simulink model "DataDrivenRotaryPendulum"  (R2024a)
settings: Solver=ode1  StartTime=0.0  StopTime=SIMULATION_TIME  FixedStep=STEP_SIZE  MaxStep=1e-2  RelTol=1e-3  EnableMultiTasking=on
values from neighbouring files (symbols this model uses):
  Tf1 = 0.08    [dd_initialization.m]
  Tf2 = 0.08    [dd_initialization.m]
undefined symbols (not defined in the file or in its folder): kP
libraries: arduinolib x6, arduinosensorlib x2, simulink x1
settings Model: ExtModeTrigDuration=2  Creator=ikumi  LastModifiedBy=Huan
settings SolverCC: AutoInsertRateTranBlk=on
settings OptimizationCC: EnhancedBackFolding=on  PassReuseOutputArgsAs=Individual arguments  ZeroExternalMemoryAtStartup=off  ZeroInternalMemoryAtStartup=off  MaxStackSize=64  OptimizeBlockOrder=speed  DifferentSizesBufferReuse=on  OptimizationCustomize=off  EfficientTunableParamExpr=on
settings DebuggingCC: ParameterTunabilityLossMsg=error
settings HardwareCC: ProdBitPerInt=16  ProdBitPerPointer=16  ProdBitPerSizeT=16  ProdBitPerPtrDiffT=16  ProdLargestAtomicFloat=None  ProdWordSize=8  ProdHWDeviceType=Atmel->AVR
settings SFSimCC: MATLABDynamicMemAlloc=off
settings RTWCC: Description=Embedded Coder  SystemTargetFile=ert.tlc  HardwareBoard=Arduino Mega 2560  TemplateMakefile=ert_default_tmf  Toolchain=Arduino AVR  BuildConfiguration=Faster Runs
settings CodeAppCC: ForceParamTrailComments=on  IgnoreCustomStorageClasses=off  OperatorAnnotations=on  SimulinkDataObjDesc=on  SFDataObjDesc=on  InsertBlockDesc=on
settings ERTTargetCC: SupportContinuousTime=on  SupportVariableSizeSignals=on  ExtModeTransport=3  ExtModeStaticAlloc=on  ExtModeAutomaticAllocSize=off  ExtModeStaticAllocSize=2048  ExtModeMexFile=ext_xcp  ExtModeIntrfLevel=Level2 - Open

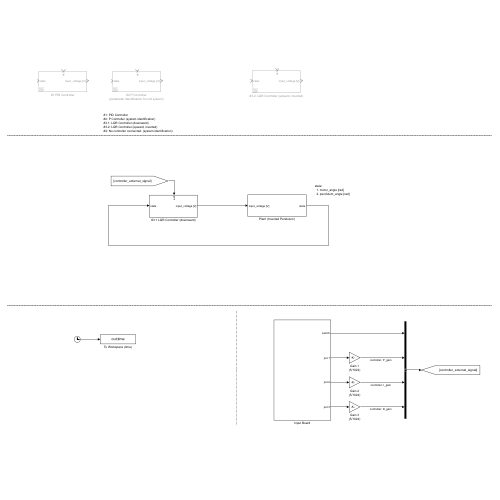
[thumbnail: Simulink's stored preview of the top-level diagram]
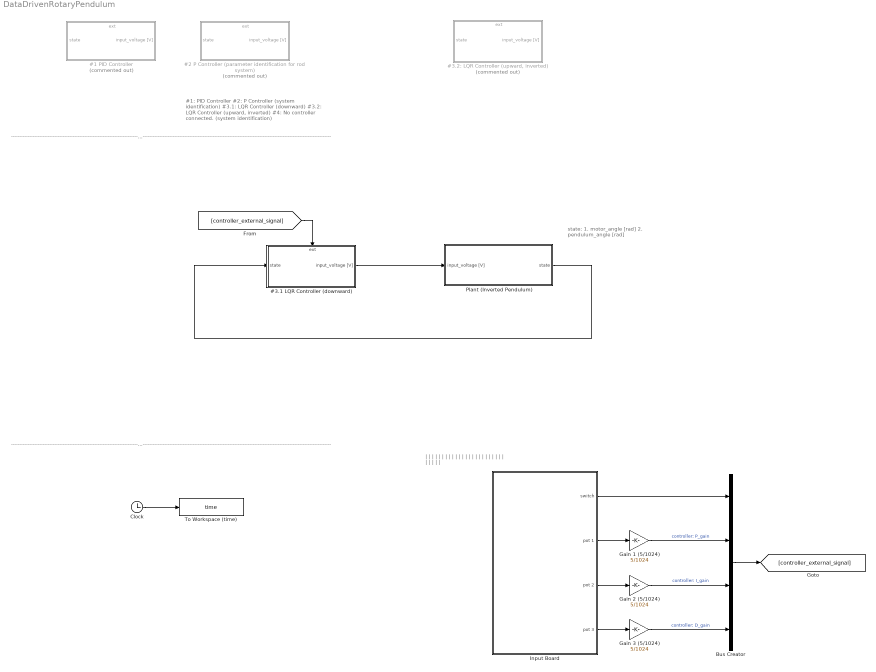
== system DataDrivenRotaryPendulum ==
  note: #1: PID Controller
      | #2: P Controller (system identification)
      | #3.1: LQR Controller (downward)
      | #3.2: LQR Controller (upward, inverted)
      | #4: No controller connected. (system identification)
  note: state:
      |   1. motor_angle [rad]
      |   2. pendulum_angle [rad]
  note: ---------------------------------------------------------------------------------------------------------------------------------------------------------------------------------------------------------------------------------------------------------------------------------------------------------------
  note: ---------------------------------------------------------------------------------------------------------------------------------------------------------------------------------------------------------------------------------------------------------------------------------------------------------------
  note: |
      | |
      | |
      | |
      | |
      | |
      | |
      | |
      | |
      | |
      | |
      | |
      | |
      | |
      | |
      | |
      | |
      | |
      | |
      | |
      | |
      | |
      | |
      | |
      | |
      | |
      | |
      | |
      | |
  #1 PID Controller : Subsystem  Commented=on
      settings: PortSchema="{\"entries\":[{\"content\":{\"sides\":[{\"content\":{\"connectorIds\":[\"In1\"]},\"type\":\"ConnectorPlacement.EquallySpacedRectSide\",\"uuid\":\"06b1af0d-78b4-43f6-add2-f1fa4860a799\"},{\"content\":{\"connectorIds\":[\"Out1\"],\"side\":\"RIGHT\"},\"type\":\"ConnectorPlacement.EquallySpacedRectSide\",\"uuid\":\"b0406211-1281-4717-b124-aa786d2c437a\"},{\"content\":{\"connectorIds\":[\"In2\"],\"side\":\"TOP\"},\"type\":\"ConnectorPlacement.EquallySpacedRectSide\",\"uuid\":\"48ff4668-84b7-46be-8f03-fa5aff98d356\"}]},\"type\":\"ConnectorPlacement.EquallySpacedConnector\",\"uuid\":\"c896c89d-b1ba-497e-85db-732d3a9a5cce\"}],\"packageUris\":[\"http://schema.mathworks.com/mf0/Connector/R2020b\"],\"version\":\"1.0\"}"
  #2 P Controller (parameter identification for rod system) : Subsystem  Commented=on
      settings: PortSchema="{\"entries\":[{\"content\":{\"sides\":[{\"content\":{\"connectorIds\":[\"In1\"]},\"type\":\"ConnectorPlacement.EquallySpacedRectSide\",\"uuid\":\"06b1af0d-78b4-43f6-add2-f1fa4860a799\"},{\"content\":{\"connectorIds\":[\"Out1\"],\"side\":\"RIGHT\"},\"type\":\"ConnectorPlacement.EquallySpacedRectSide\",\"uuid\":\"b0406211-1281-4717-b124-aa786d2c437a\"},{\"content\":{\"connectorIds\":[\"In2\"],\"side\":\"TOP\"},\"type\":\"ConnectorPlacement.EquallySpacedRectSide\",\"uuid\":\"48ff4668-84b7-46be-8f03-fa5aff98d356\"}]},\"type\":\"ConnectorPlacement.EquallySpacedConnector\",\"uuid\":\"c896c89d-b1ba-497e-85db-732d3a9a5cce\"}],\"packageUris\":[\"http://schema.mathworks.com/mf0/Connector/R2020b\"],\"version\":\"1.0\"}"
  #3.1 LQR Controller (downward) : Subsystem
      settings: PortSchema="{\"entries\":[{\"content\":{\"sides\":[{\"content\":{\"connectorIds\":[\"In1\"]},\"type\":\"ConnectorPlacement.EquallySpacedRectSide\",\"uuid\":\"b3e4cd4f-c8f8-4ac1-a1f2-23e37a640ad8\"},{\"content\":{\"connectorIds\":[\"Out1\"],\"side\":\"RIGHT\"},\"type\":\"ConnectorPlacement.EquallySpacedRectSide\",\"uuid\":\"02360ac2-7779-4092-8f90-91424c435481\"},{\"content\":{\"connectorIds\":[\"In2\"],\"side\":\"TOP\"},\"type\":\"ConnectorPlacement.EquallySpacedRectSide\",\"uuid\":\"f86ccd1f-d9a7-4ad2-ba4f-ea0c1bd32c00\"}]},\"type\":\"ConnectorPlacement.EquallySpacedConnector\",\"uuid\":\"875a99af-631d-422d-8b23-87ab8d1e3283\"}],\"packageUris\":[\"http://schema.mathworks.com/mf0/Connector/R2020b\"],\"version\":\"1.0\"}"
  "#3.2: LQR Controller (upward, inverted)" : Subsystem  Commented=on
      settings: PortSchema="{\"entries\":[{\"content\":{\"sides\":[{\"content\":{\"connectorIds\":[\"In1\"]},\"type\":\"ConnectorPlacement.EquallySpacedRectSide\",\"uuid\":\"b3e4cd4f-c8f8-4ac1-a1f2-23e37a640ad8\"},{\"content\":{\"connectorIds\":[\"Out1\"],\"side\":\"RIGHT\"},\"type\":\"ConnectorPlacement.EquallySpacedRectSide\",\"uuid\":\"02360ac2-7779-4092-8f90-91424c435481\"},{\"content\":{\"connectorIds\":[\"In2\"],\"side\":\"TOP\"},\"type\":\"ConnectorPlacement.EquallySpacedRectSide\",\"uuid\":\"f86ccd1f-d9a7-4ad2-ba4f-ea0c1bd32c00\"}]},\"type\":\"ConnectorPlacement.EquallySpacedConnector\",\"uuid\":\"875a99af-631d-422d-8b23-87ab8d1e3283\"}],\"packageUris\":[\"http://schema.mathworks.com/mf0/Connector/R2020b\"],\"version\":\"1.0\"}"
  Bus Creator : BusCreator  Inputs=4
  Clock : Clock
  Gain 1 (5/1024) : Gain  Gain=5/1024
  Gain 2 (5/1024) : Gain  Gain=5/1024
  Gain 3 (5/1024) : Gain  Gain=5/1024
  Input Board : Subsystem
  Plant (Inverted Pendulum) : Subsystem
  To Workspace (time) : ToWorkspace  VariableName=time  SaveFormat=Timeseries  SampleTime=-1
  wires:
  #3.1 LQR Controller (downward)/1(input_voltage [V]) -> Plant (Inverted Pendulum)/1(input_voltage [V])
  Input Board/1(switch) -> Bus Creator/1
  Gain 2 (5/1024)/1 -> Bus Creator/3  "controller: I_gain"
  Input Board/4(pot 3) -> Gain 3 (5/1024)/1
  Gain 1 (5/1024)/1 -> Bus Creator/2  "controller: P_gain"
  Gain 3 (5/1024)/1 -> Bus Creator/4  "controller: D_gain"
  Input Board/3(pot 2) -> Gain 2 (5/1024)/1
  Input Board/2(pot 1) -> Gain 1 (5/1024)/1
  Bus Creator/1 -> [controller_external_signal]
  [controller_external_signal] -> #3.1 LQR Controller (downward)/2(ext)
  Clock/1 -> To Workspace (time)/1
  Plant (Inverted Pendulum)/1(state) -> #3.1 LQR Controller (downward)/1(state)

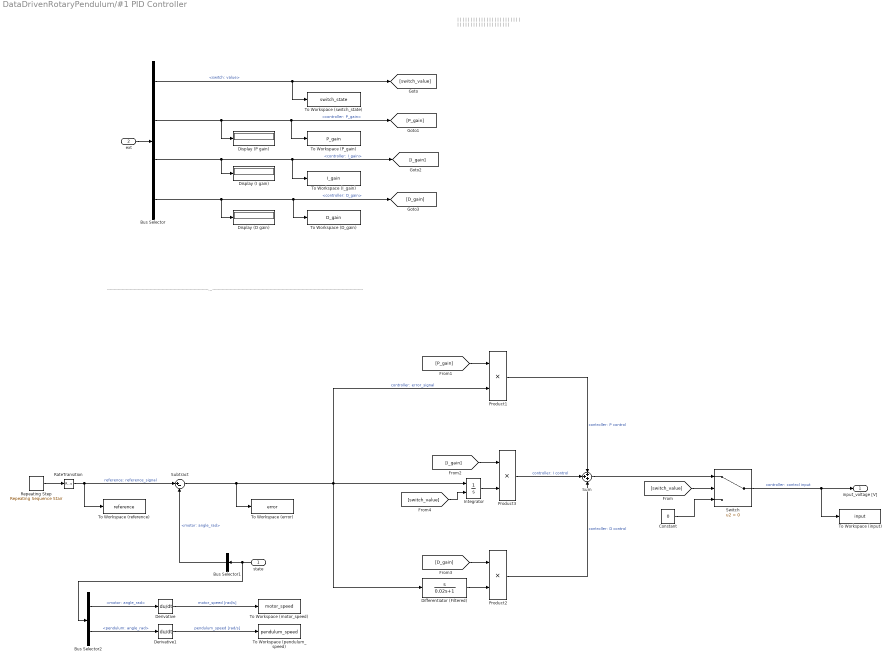
== system DataDrivenRotaryPendulum/#1 PID Controller ==
  note: ---------------------------------------------------------------------------------------------------------------------------------------------------------------------------------------------------------------------------------------------------------------------------------------------------------------
  note: |
      | |
      | |
      | |
      | |
      | |
      | |
      | |
      | |
      | |
      | |
      | |
      | |
      | |
      | |
      | |
      | |
      | |
      | |
      | |
      | |
      | |
      | |
      | |
      | |
      | |
      | |
      | |
      | |
      | |
      | |
      | |
      | |
      | |
      | |
      | |
      | |
      | |
      | |
      | |
      | |
      | |
      | |
      | |
  state : Inport
  ext : Inport  Port=2
  " Integrator " : Integrator  ExternalReset=rising
  Bus Selector : BusSelector  OutputSignals=switch: value,controller: P_gain,controller: I_gain,controller: D_gain
  Bus Selector1 : BusSelector  OutputSignals=motor: angle_rad
  Bus Selector2 : BusSelector  OutputSignals=motor: angle_rad,pendulum: angle_rad
  Constant : Constant  Value=0
  Derivative : Derivative
  Derivative1 : Derivative
  Differentiator (Filtered) : TransferFcn  Numerator=[1 0]  Denominator=[0.02 1]
  Display (D gain) : Display
  Display (I gain) : Display
  Display (P gain) : Display
  Product1 : Product
  Product2 : Product
  Product3 : Product
  RateTransition : RateTransition  OutPortSampleTime=STEP_SIZE
  Repeating Step : simulink/Sources/Repeating Sequence Stair  OutValues=[pi/2 0 -pi/2 0]  tsamp=2.5  OutMin=[]  OutMax=[]  OutDataTypeStr=double  OutputDataTypeScalingMode=double  OutDataType=fixdt(0,8)  ConRadixGroup=Best Precision: Vector-wise  OutScaling=2^-12
  Subtract : Sum  Inputs=|+-
  Sum : Sum  Inputs=+++
  Switch : Switch  Criteria=u2 > Threshold  SaturateOnIntegerOverflow=off  InputSameDT=off
  To Workspace (D_gain) : ToWorkspace  VariableName=D_gain  SaveFormat=Timeseries  SampleTime=-1
  To Workspace (I_gain) : ToWorkspace  VariableName=I_gain  SaveFormat=Timeseries  SampleTime=-1
  To Workspace (P_gain) : ToWorkspace  VariableName=P_gain  SaveFormat=Timeseries  SampleTime=-1
  To Workspace (error) : ToWorkspace  VariableName=error  SaveFormat=Timeseries  SampleTime=-1
  To Workspace (input) : ToWorkspace  VariableName=input  SaveFormat=Timeseries  SampleTime=-1
  To Workspace (motor_speed) : ToWorkspace  VariableName=motor_speed  SaveFormat=Timeseries  SampleTime=-1
  To Workspace (pendulum_speed) : ToWorkspace  VariableName=pendulum_speed  SaveFormat=Timeseries  SampleTime=-1
  To Workspace (reference) : ToWorkspace  VariableName=reference  SaveFormat=Timeseries  SampleTime=-1
  To Workspace (switch_state) : ToWorkspace  VariableName=switch_state  SaveFormat=Timeseries  SampleTime=-1
  input_voltage [V] : Outport
  wires:
  Constant/1 -> Switch/3
  Subtract/1 -> To Workspace (error)/1, Differentiator (Filtered)/1, " Integrator "/1, Product1/2  "controller: error_signal"
  [P_gain] -> Product1/1
  [I_gain] -> Product3/1
  [D_gain] -> Product2/1
  " Integrator "/1 -> Product3/2
  Differentiator (Filtered)/1 -> Product2/2
  Product3/1 -> Sum/2  "controller: I control"
  Product2/1 -> Sum/3  "controller: D control"
  Product1/1 -> Sum/1  "controller: P control"
  Sum/1 -> Switch/1
  [switch_value] -> Switch/2
  Switch/1 -> To Workspace (input)/1, input_voltage [V]/1  "controller: control input"
  [switch_value] -> " Integrator "/2
  Bus Selector/3 -> To Workspace (I_gain)/1, [I_gain], Display (I gain)/1  "<controller: I_gain>"
  Bus Selector/4 -> To Workspace (D_gain)/1, [D_gain], Display (D gain)/1  "<controller: D_gain>"
  Bus Selector/1 -> To Workspace (switch_state)/1, [switch_value]  "<switch: value>"
  Bus Selector/2 -> To Workspace (P_gain)/1, [P_gain], Display (P gain)/1  "<controller: P_gain>"
  ext/1 -> Bus Selector/1
  Repeating Step/1 -> RateTransition/1
  RateTransition/1 -> Subtract/1, To Workspace (reference)/1  "reference: reference_signal"
  Bus Selector1/1 -> Subtract/2  "<motor: angle_rad>"
  Bus Selector2/2 -> Derivative1/1  "<pendulum: angle_rad>"
  Derivative1/1 -> To Workspace (pendulum_speed)/1  "pendulum_speed [rad/s]"
  state/1 -> Bus Selector2/1, Bus Selector1/1
  Bus Selector2/1 -> Derivative/1  "<motor: angle_rad>"
  Derivative/1 -> To Workspace (motor_speed)/1  "motor_speed [rad/s]"

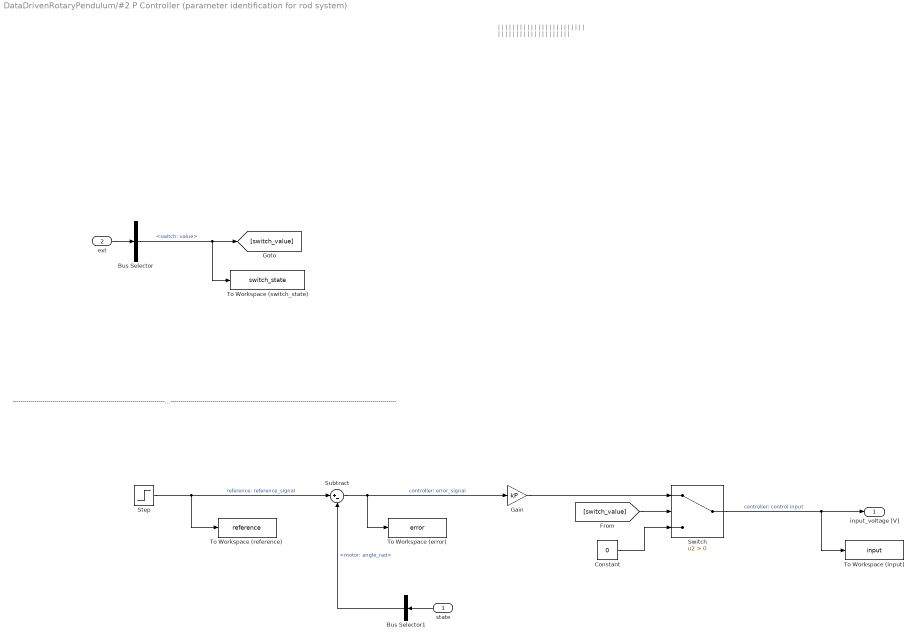
== system DataDrivenRotaryPendulum/#2 P Controller (parameter identification for rod system) ==
  note: ---------------------------------------------------------------------------------------------------------------------------------------------------------------------------------------------------------------------------------------------------------------------------------------------------------------
  note: |
      | |
      | |
      | |
      | |
      | |
      | |
      | |
      | |
      | |
      | |
      | |
      | |
      | |
      | |
      | |
      | |
      | |
      | |
      | |
      | |
      | |
      | |
      | |
      | |
      | |
      | |
      | |
      | |
      | |
      | |
      | |
      | |
      | |
      | |
      | |
      | |
      | |
      | |
      | |
      | |
      | |
      | |
      | |
  state : Inport
  ext : Inport  Port=2
  Bus Selector : BusSelector  OutputSignals=switch: value
  Bus Selector1 : BusSelector  OutputSignals=motor: angle_rad
  Constant : Constant  Value=0
  Gain : Gain  Gain=kP
  Step : Step  After=pi/2  SampleTime=0
  Subtract : Sum  Inputs=|+-
  Switch : Switch  Criteria=u2 > Threshold  SaturateOnIntegerOverflow=off  InputSameDT=off
  To Workspace (error) : ToWorkspace  VariableName=error  SaveFormat=Timeseries  SampleTime=-1
  To Workspace (input) : ToWorkspace  VariableName=input  SaveFormat=Timeseries  SampleTime=-1
  To Workspace (reference) : ToWorkspace  VariableName=reference  SaveFormat=Timeseries  SampleTime=-1
  To Workspace (switch_state) : ToWorkspace  VariableName=switch_state  SaveFormat=Timeseries  SampleTime=-1
  input_voltage [V] : Outport
  wires:
  Constant/1 -> Switch/3
  Subtract/1 -> Gain/1, To Workspace (error)/1  "controller: error_signal"
  Gain/1 -> Switch/1
  [switch_value] -> Switch/2
  Switch/1 -> To Workspace (input)/1, input_voltage [V]/1  "controller: control input"
  Bus Selector/1 -> [switch_value], To Workspace (switch_state)/1  "<switch: value>"
  ext/1 -> Bus Selector/1
  Step/1 -> Subtract/1, To Workspace (reference)/1  "reference: reference_signal"
  state/1 -> Bus Selector1/1
  Bus Selector1/1 -> Subtract/2  "<motor: angle_rad>"

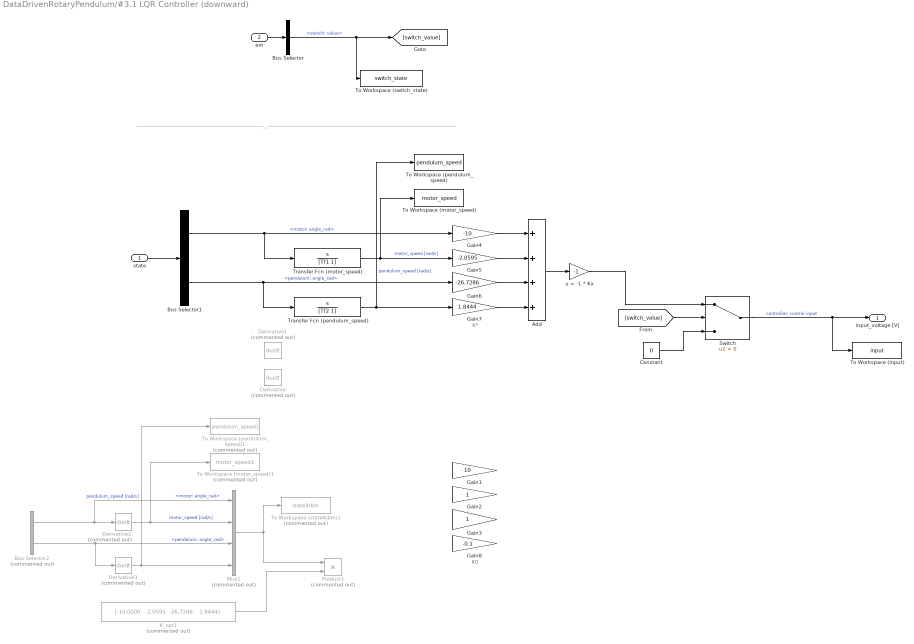
== system DataDrivenRotaryPendulum/#3.1 LQR Controller (downward) ==
  note: ---------------------------------------------------------------------------------------------------------------------------------------------------------------------------------------------------------------------------------------------------------------------------------------------------------------
  note: K*
  note: K0
  state : Inport
  ext : Inport  Port=2
  Add : Sum  Inputs=++++
  Bus Selector : BusSelector  OutputSignals=switch: value
  Bus Selector1 : BusSelector  OutputSignals=motor: angle_rad,pendulum: angle_rad
  Bus Selector2 : BusSelector  Commented=on  OutputSignals=motor: angle_rad,pendulum: angle_rad
  Constant : Constant  Value=0
  Derivative{,1..3} (4 alike) : Derivative  Commented=on
  Gain1 : Gain  Gain=10
  Gain2 : Gain
  Gain3 : Gain
  Gain4 : Gain  Gain=-10
  Gain5 : Gain  Gain=-2.0595
  Gain6 : Gain  Gain=-26.7286
  Gain7 : Gain  Gain=1.8444
  Gain8 : Gain  Gain=-0.1
  K_opt1 : Constant  Commented=on  Value="[-10.0000   -2.0595  -26.7286    1.8444]"
  Mux1 : Mux  Commented=on
  Product1 : Product  Commented=on
  Switch : Switch  Criteria=u2 > Threshold  SaturateOnIntegerOverflow=off  InputSameDT=off
  To Workspace (input) : ToWorkspace  VariableName=input  SaveFormat=Timeseries  SampleTime=-1
  To Workspace (motor_speed) : ToWorkspace  VariableName=motor_speed  SaveFormat=Timeseries  SampleTime=-1
  To Workspace (motor_speed)1 : ToWorkspace  Commented=on  VariableName=motor_speed1  SaveFormat=Timeseries  SampleTime=-1
  To Workspace (pendulum_speed) : ToWorkspace  VariableName=pendulum_speed  SaveFormat=Timeseries  SampleTime=-1
  To Workspace (pendulum_speed)1 : ToWorkspace  Commented=on  VariableName=pendulum_speed1  SaveFormat=Timeseries  SampleTime=-1
  To Workspace (state4dim)1 : ToWorkspace  Commented=on  VariableName=state4dim  SaveFormat=Timeseries  SampleTime=-1
  To Workspace (switch_state) : ToWorkspace  VariableName=switch_state  SaveFormat=Timeseries  SampleTime=-1
  "Transfer Fcn (motor_speed) " : TransferFcn  Numerator=[1 0]  Denominator=[Tf1 1]
  Transfer Fcn (pendulum_speed) : TransferFcn  Numerator=[1 0]  Denominator=[Tf2 1]
  u = -1 * Kx : Gain  Gain=-1
  input_voltage [V] : Outport
  wires:
  Constant/1 -> Switch/3
  [switch_value] -> Switch/2
  Switch/1 -> To Workspace (input)/1, input_voltage [V]/1  "controller: control input"
  state/1 -> Bus Selector1/1
  Bus Selector1/1 -> Gain4/1, "Transfer Fcn (motor_speed) "/1  "<motor: angle_rad>"
  Bus Selector1/2 -> Gain6/1, Transfer Fcn (pendulum_speed)/1  "<pendulum: angle_rad>"
  "Transfer Fcn (motor_speed) "/1 -> Gain5/1, To Workspace (motor_speed)/1  "motor_speed [rad/s]"
  Transfer Fcn (pendulum_speed)/1 -> Gain7/1, To Workspace (pendulum_speed)/1  "pendulum_speed [rad/s]"
  Add/1 -> u = -1 * Kx/1
  Bus Selector/1 -> [switch_value], To Workspace (switch_state)/1  "<switch: value>"
  ext/1 -> Bus Selector/1
  Bus Selector2/2 -> Derivative3/1, Mux1/3  "<pendulum: angle_rad>"
  Mux1/1 -> To Workspace (state4dim)1/1, Product1/1
  Derivative3/1 -> To Workspace (pendulum_speed)1/1, Mux1/4  "pendulum_speed [rad/s]"
  K_opt1/1 -> Product1/2
  Bus Selector2/1 -> Mux1/1, Derivative2/1  "<motor: angle_rad>"
  Derivative2/1 -> To Workspace (motor_speed)1/1, Mux1/2  "motor_speed [rad/s]"
  Gain4/1 -> Add/1
  Gain5/1 -> Add/2
  Gain6/1 -> Add/3
  Gain7/1 -> Add/4
  u = -1 * Kx/1 -> Switch/1

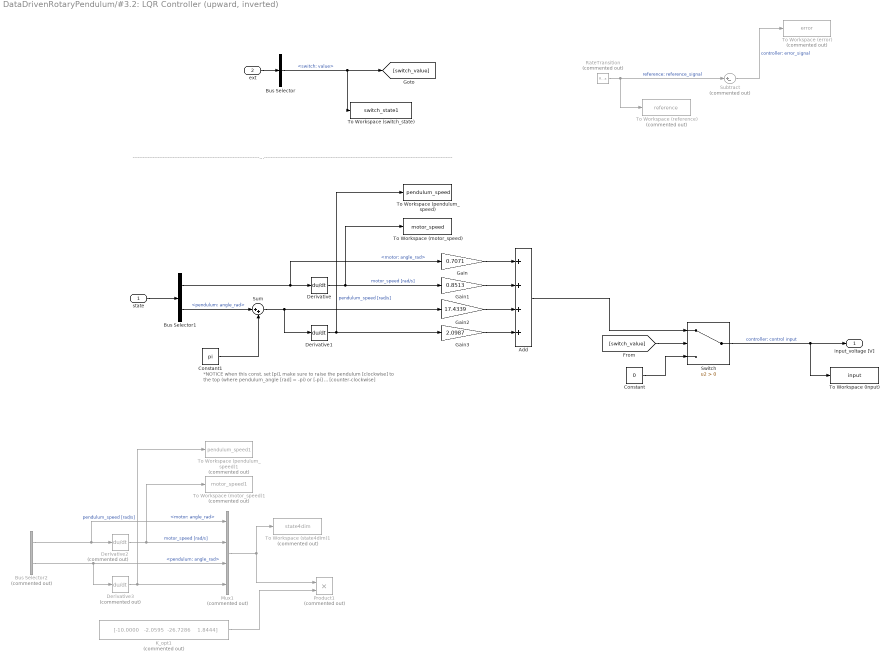
== system DataDrivenRotaryPendulum/#3.2: LQR Controller (upward, inverted) ==
  note: *NOTICE
      | when this const. set [pi], make sure to
      | raise the pendulum [clockwise] to the top (where pendulum_angle [rad] = -pi)
      | or [-pi] ... [counter-clockwise]
  note: ---------------------------------------------------------------------------------------------------------------------------------------------------------------------------------------------------------------------------------------------------------------------------------------------------------------
  state : Inport
  ext : Inport  Port=2
  Add : Sum  Inputs=++++
  Bus Selector : BusSelector  OutputSignals=switch: value
  Bus Selector1 : BusSelector  OutputSignals=motor: angle_rad,pendulum: angle_rad
  Bus Selector2 : BusSelector  Commented=on  OutputSignals=motor: angle_rad,pendulum: angle_rad
  Constant : Constant  Value=0
  Constant1 : Constant  Value=pi
  Derivative : Derivative
  Derivative1 : Derivative
  Derivative2 : Derivative  Commented=on
  Derivative3 : Derivative  Commented=on
  Gain : Gain  Gain=0.7071
  Gain1 : Gain  Gain=0.8513
  Gain2 : Gain  Gain=17.4339
  Gain3 : Gain  Gain=2.0987
  K_opt1 : Constant  Commented=on  Value="[-10.0000   -2.0595  -26.7286    1.8444]"
  Mux1 : Mux  Commented=on
  Product1 : Product  Commented=on
  RateTransition : RateTransition  Commented=on  OutPortSampleTime=STEP_SIZE
  Subtract : Sum  Commented=on  Inputs=|+-
  Sum : Sum  Inputs=|++
  Switch : Switch  Criteria=u2 > Threshold  SaturateOnIntegerOverflow=off  InputSameDT=off
  To Workspace (error) : ToWorkspace  Commented=on  VariableName=error  SaveFormat=Timeseries  SampleTime=-1
  To Workspace (input) : ToWorkspace  VariableName=input  SaveFormat=Timeseries  SampleTime=-1
  To Workspace (motor_speed) : ToWorkspace  VariableName=motor_speed  SaveFormat=Timeseries  SampleTime=-1
  To Workspace (motor_speed)1 : ToWorkspace  Commented=on  VariableName=motor_speed1  SaveFormat=Timeseries  SampleTime=-1
  To Workspace (pendulum_speed) : ToWorkspace  VariableName=pendulum_speed  SaveFormat=Timeseries  SampleTime=-1
  To Workspace (pendulum_speed)1 : ToWorkspace  Commented=on  VariableName=pendulum_speed1  SaveFormat=Timeseries  SampleTime=-1
  To Workspace (reference) : ToWorkspace  Commented=on  VariableName=reference  SaveFormat=Timeseries  SampleTime=-1
  To Workspace (state4dim)1 : ToWorkspace  Commented=on  VariableName=state4dim  SaveFormat=Timeseries  SampleTime=-1
  To Workspace (switch_state) : ToWorkspace  VariableName=switch_state1  SaveFormat=Timeseries  SampleTime=-1
  input_voltage [V] : Outport
  wires:
  Sum/1 -> Gain2/1, Derivative1/1
  Constant1/1 -> Sum/2
  Gain3/1 -> Add/4
  Gain2/1 -> Add/3
  Gain1/1 -> Add/2
  Gain/1 -> Add/1
  Derivative2/1 -> Mux1/2, To Workspace (motor_speed)1/1  "motor_speed [rad/s]"
  Bus Selector2/1 -> Derivative2/1, Mux1/1  "<motor: angle_rad>"
  K_opt1/1 -> Product1/2
  Derivative3/1 -> Mux1/4, To Workspace (pendulum_speed)1/1  "pendulum_speed [rad/s]"
  Mux1/1 -> Product1/1, To Workspace (state4dim)1/1
  Bus Selector2/2 -> Mux1/3, Derivative3/1  "<pendulum: angle_rad>"
  ext/1 -> Bus Selector/1
  Bus Selector/1 -> To Workspace (switch_state)/1, [switch_value]  "<switch: value>"
  Add/1 -> Switch/1
  Derivative1/1 -> Gain3/1, To Workspace (pendulum_speed)/1  "pendulum_speed [rad/s]"
  Derivative/1 -> Gain1/1, To Workspace (motor_speed)/1  "motor_speed [rad/s]"
  Bus Selector1/2 -> Sum/1  "<pendulum: angle_rad>"
  Bus Selector1/1 -> Gain/1, Derivative/1  "<motor: angle_rad>"
  state/1 -> Bus Selector1/1
  RateTransition/1 -> To Workspace (reference)/1, Subtract/1  "reference: reference_signal"
  Switch/1 -> input_voltage [V]/1, To Workspace (input)/1  "controller: control input"
  [switch_value] -> Switch/2
  Subtract/1 -> To Workspace (error)/1  "controller: error_signal"
  Constant/1 -> Switch/3

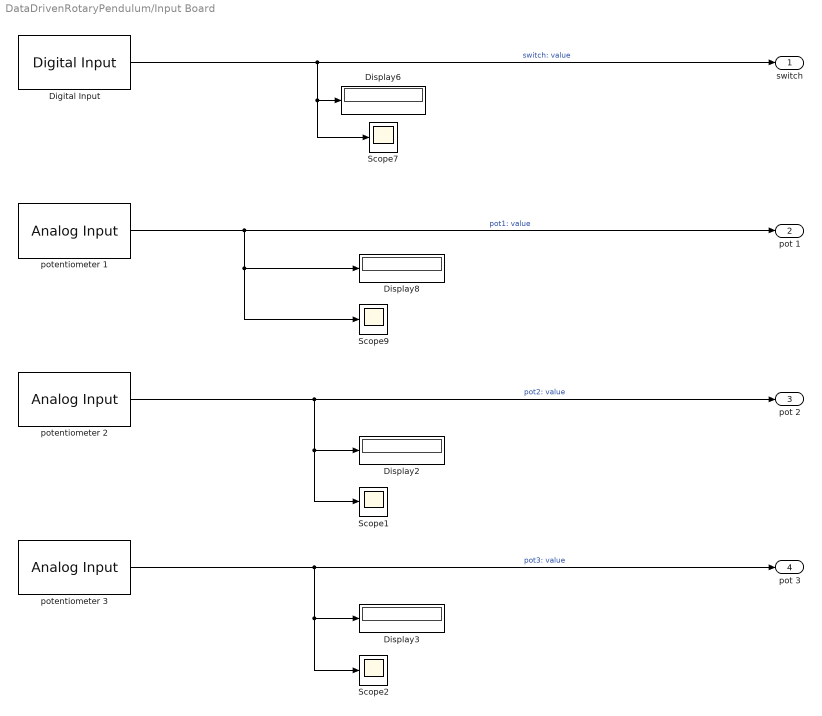
== system DataDrivenRotaryPendulum/Input Board ==
  Digital Input : arduinolib/Digital Input  pinNumber=8  mode=Default  Direction=input  SampleTime=-1  blockPlatform=arduino
  Display{2..3,6,8} (4 alike) : Display
  Scope{1..2,7,9} (4 alike) : Scope
  potentiometer 1 : arduinolib/Analog Input  pinNumber=0  ReadResultsOnly=off  ConversionTriggerSource=Software  ExternalTriggerType=uint32( 0 )  OutputDataType=uint16  EnableConversionCompleteNotify=off  EnableOuputStatus=off  SampleTime=-1  blockPlatform=arduino
  potentiometer 2 : arduinolib/Analog Input  pinNumber=1  ReadResultsOnly=off  ConversionTriggerSource=Software  ExternalTriggerType=uint32( 0 )  OutputDataType=uint16  EnableConversionCompleteNotify=off  EnableOuputStatus=off  SampleTime=-1  blockPlatform=arduino
  potentiometer 3 : arduinolib/Analog Input  pinNumber=2  ReadResultsOnly=off  ConversionTriggerSource=Software  ExternalTriggerType=uint32( 0 )  OutputDataType=uint16  EnableConversionCompleteNotify=off  EnableOuputStatus=off  SampleTime=-1  blockPlatform=arduino
  switch : Outport
  pot 1 : Outport  Port=2
  pot 2 : Outport  Port=3
  pot 3 : Outport  Port=4
  wires:
  Digital Input/1 -> switch/1, Scope7/1, Display6/1  "switch: value"
  potentiometer 3/1 -> pot 3/1, Scope2/1, Display3/1  "pot3: value"
  potentiometer 2/1 -> pot 2/1, Scope1/1, Display2/1  "pot2: value"
  potentiometer 1/1 -> Scope9/1, Display8/1, pot 1/1  "pot1: value"

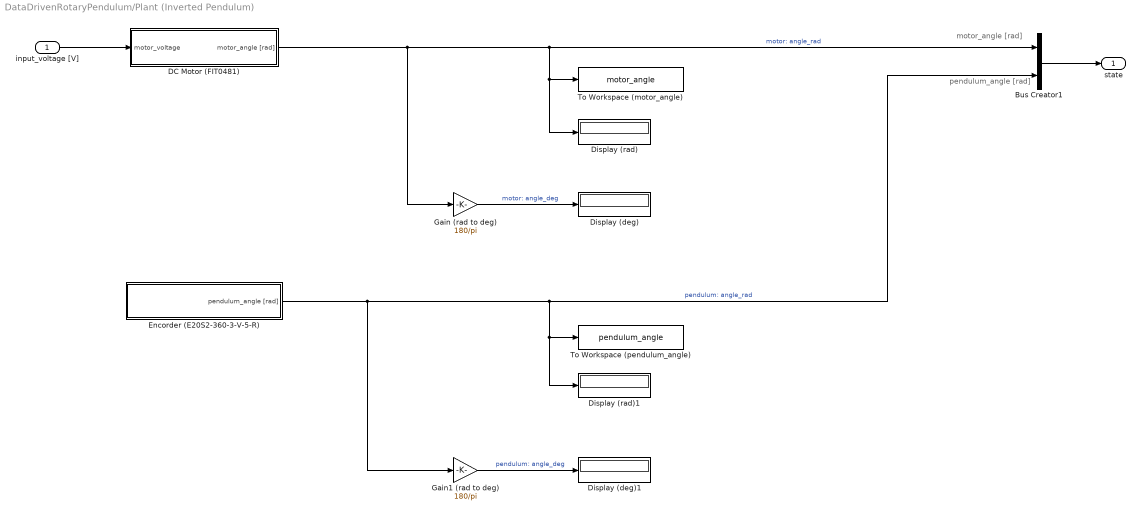
== system DataDrivenRotaryPendulum/Plant (Inverted Pendulum) ==
  note: pendulum_angle [rad]
  note: motor_angle [rad]
  input_voltage [V] : Inport
  Bus Creator1 : BusCreator  Inputs=2
  DC Motor (FIT0481) : Subsystem
  Display (deg) : Display
  Display (deg)1 : Display
  Display (rad) : Display
  Display (rad)1 : Display
  Encorder (E20S2-360-3-V-5-R) : Subsystem
  Gain (rad to deg) : Gain  Gain=180/pi
  Gain1 (rad to deg) : Gain  Gain=180/pi
  To Workspace (motor_angle) : ToWorkspace  VariableName=motor_angle  SaveFormat=Timeseries  SampleTime=-1
  To Workspace (pendulum_angle) : ToWorkspace  VariableName=pendulum_angle  SaveFormat=Timeseries  SampleTime=-1
  state : Outport
  wires:
  DC Motor (FIT0481)/1(motor_angle [rad]) -> To Workspace (motor_angle)/1, Display (rad)/1, Bus Creator1/1, Gain (rad to deg)/1  "motor: angle_rad"
  Gain (rad to deg)/1 -> Display (deg)/1  "motor: angle_deg"
  input_voltage [V]/1 -> DC Motor (FIT0481)/1(motor_voltage)
  Encorder (E20S2-360-3-V-5-R)/1(pendulum_angle [rad]) -> Bus Creator1/2, To Workspace (pendulum_angle)/1, Display (rad)1/1, Gain1 (rad to deg)/1  "pendulum: angle_rad"
  Gain1 (rad to deg)/1 -> Display (deg)1/1  "pendulum: angle_deg"
  Bus Creator1/1 -> state/1

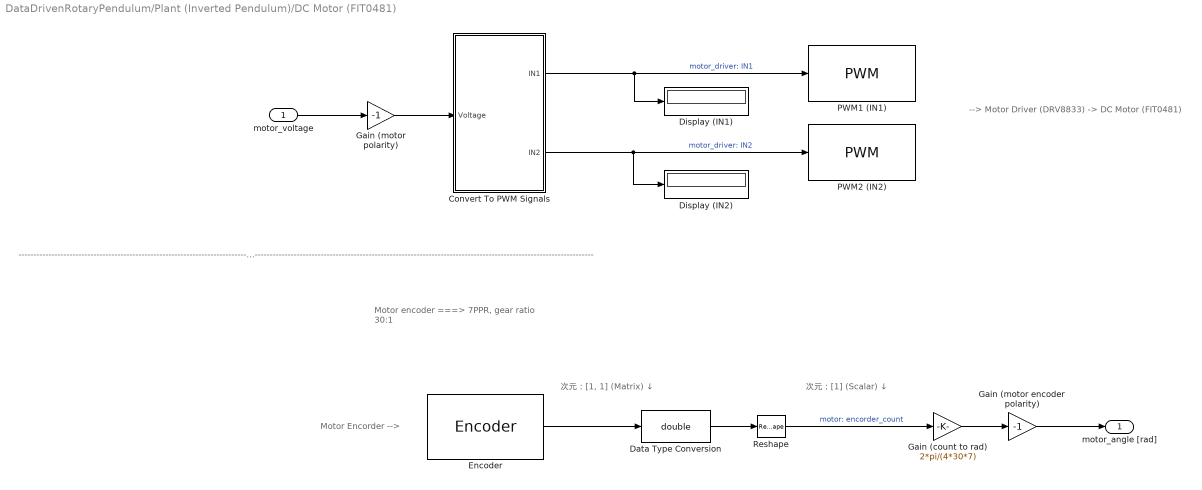
== system DataDrivenRotaryPendulum/Plant (Inverted Pendulum)/DC Motor (FIT0481) ==
  note: Motor Encorder -->
  note: --> Motor Driver (DRV8833) -> DC Motor (FIT0481)
  note: Motor encoder
      | ===> 7PPR, gear ratio 30:1
  note: 次元：[1, 1] (Matrix)
      | ↓
  note: 次元：[1] (Scalar)
      | ↓
  note: ---------------------------------------------------------------------------------------------------------------------------------------------------------------------------------------------------------------------------------------------------------------------------------------------------------------
  motor_voltage : Inport
  Convert To PWM Signals : Subsystem
  Data Type Conversion : DataTypeConversion  OutDataTypeStr=double  SaturateOnIntegerOverflow=off  RndMeth=Floor
  Display (IN1) : Display
  Display (IN2) : Display
  Encoder : arduinosensorlib/Encoder  InputA=2  InputB=3  Mode=No reset  SampleTime=-1
  Gain (count to rad) : Gain  Gain=2*pi/(4*30*7)
  Gain (motor encoder polarity) : Gain  Gain=-1
  Gain (motor polarity) : Gain  Gain=-1
  PWM1 (IN1) : arduinolib/PWM  pinNumber=6  frequencyType=Default  desiredFrequency=490.2  achievableFrequency=490.2
  PWM2 (IN2) : arduinolib/PWM  pinNumber=7  frequencyType=Default  desiredFrequency=490.2  achievableFrequency=490.2
  Reshape : Reshape
  motor_angle [rad] : Outport
  wires:
  Gain (motor polarity)/1 -> Convert To PWM Signals/1(Voltage)
  Convert To PWM Signals/1(IN1) -> Display (IN1)/1, PWM1 (IN1)/1  "motor_driver: IN1"
  Convert To PWM Signals/2(IN2) -> Display (IN2)/1, PWM2 (IN2)/1  "motor_driver: IN2"
  Encoder/1 -> Data Type Conversion/1
  Gain (count to rad)/1 -> Gain (motor encoder polarity)/1
  Reshape/1 -> Gain (count to rad)/1  "motor: encorder_count"
  Data Type Conversion/1 -> Reshape/1
  Gain (motor encoder polarity)/1 -> motor_angle [rad]/1
  motor_voltage/1 -> Gain (motor polarity)/1

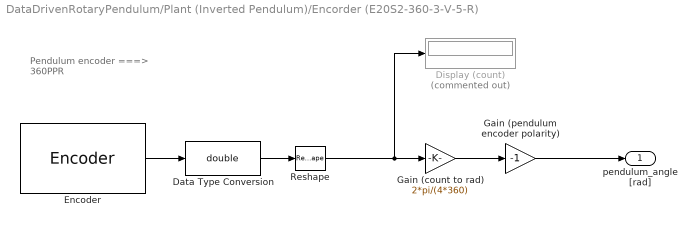
== system DataDrivenRotaryPendulum/Plant (Inverted Pendulum)/Encorder (E20S2-360-3-V-5-R) ==
  note: Pendulum encoder
      | ===> 360PPR
  Data Type Conversion : DataTypeConversion  OutDataTypeStr=double  SaturateOnIntegerOverflow=off  RndMeth=Floor
  Display (count) : Display  Commented=on
  Encoder : arduinosensorlib/Encoder  InputA=18  InputB=19  Mode=No reset  SampleTime=-1
  Gain (count to rad) : Gain  Gain=2*pi/(4*360)
  Gain (pendulum encoder polarity) : Gain  Gain=-1
  Reshape : Reshape
  pendulum_angle [rad] : Outport
  wires:
  Data Type Conversion/1 -> Reshape/1
  Reshape/1 -> Display (count)/1, Gain (count to rad)/1
  Gain (pendulum encoder polarity)/1 -> pendulum_angle [rad]/1
  Gain (count to rad)/1 -> Gain (pendulum encoder polarity)/1
  Encoder/1 -> Data Type Conversion/1

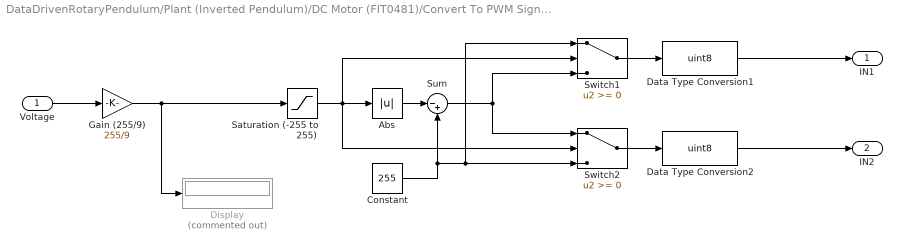
== system DataDrivenRotaryPendulum/Plant (Inverted Pendulum)/DC Motor (FIT0481)/Convert To PWM Signals ==
  Voltage : Inport
  Abs : Abs  SaturateOnIntegerOverflow=off
  Constant : Constant  Value=255  SampleTime=-1
  Data Type Conversion1 : DataTypeConversion  OutDataTypeStr=uint8  SaturateOnIntegerOverflow=off  RndMeth=Floor
  Data Type Conversion2 : DataTypeConversion  OutDataTypeStr=uint8  SaturateOnIntegerOverflow=off  RndMeth=Floor
  Display : Display  Commented=on
  Gain (255/9) : Gain  Gain=255/9
  Saturation (-255 to 255) : Saturate  UpperLimit=255  LowerLimit=-255
  Sum : Sum  Inputs=|-+
  Switch1 : Switch  SaturateOnIntegerOverflow=off  InputSameDT=off
  Switch2 : Switch  SaturateOnIntegerOverflow=off  InputSameDT=off
  IN1 : Outport
  IN2 : Outport  Port=2
  wires:
  Gain (255/9)/1 -> Display/1, Saturation (-255 to 255)/1
  Voltage/1 -> Gain (255/9)/1
  Abs/1 -> Sum/1
  Sum/1 -> Switch2/1, Switch1/3
  Switch2/1 -> Data Type Conversion2/1
  Constant/1 -> Sum/2, Switch1/1, Switch2/3
  Saturation (-255 to 255)/1 -> Abs/1, Switch1/2, Switch2/2
  Switch1/1 -> Data Type Conversion1/1
  Data Type Conversion1/1 -> IN1/1
  Data Type Conversion2/1 -> IN2/1
